simulink model "leadcar_stationary_egocar_move"  (R2025b)
settings: Solver=VariableStepAuto  StartTime=0.0  StopTime=10.0  RelTol=1e-3
settings Model: Creator=jdcjd  LastModifiedBy=jdcjd

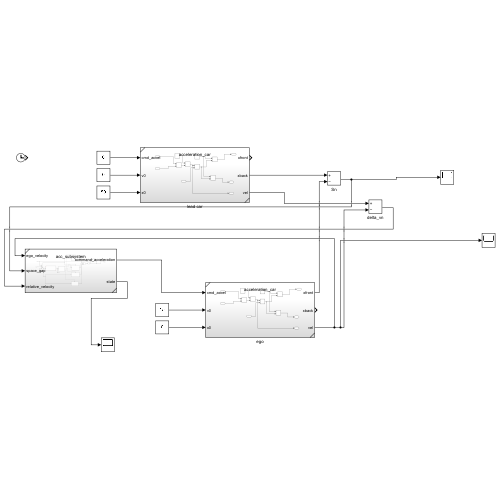
[thumbnail: Simulink's stored preview of the top-level diagram]
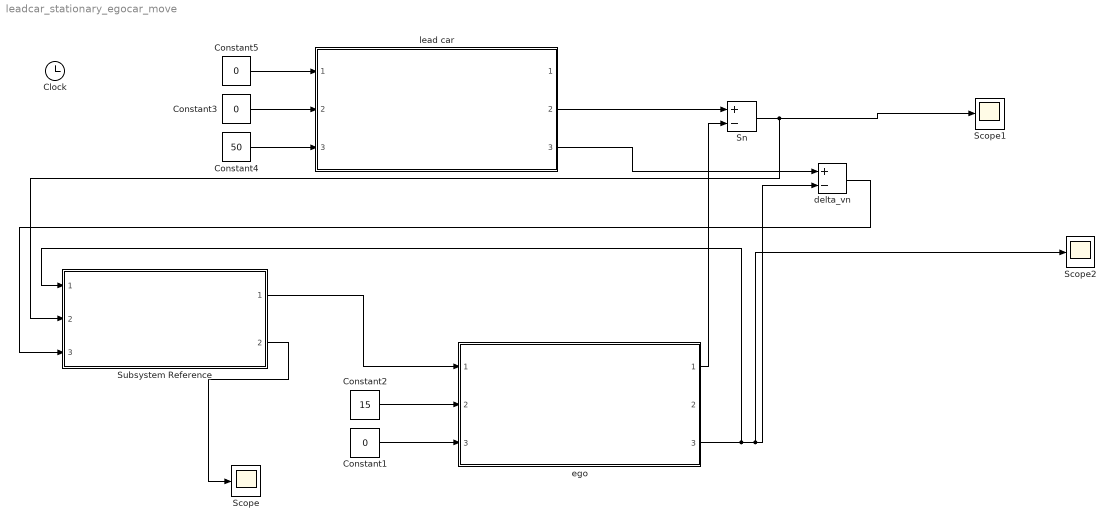
== system leadcar_stationary_egocar_move ==
  Clock : Clock
  Constant1 : Constant  Value=0
  Constant2 : Constant  Value=15
  Constant3 : Constant  Value=0
  Constant4 : Constant  Value=50
  Constant5 : Constant  Value=0
  Scope : Scope
  Scope1 : Scope
  Scope2 : Scope
      settings: DataLoggingVariableName=ScopeData2
  Sn : Sum  Inputs=+-
  Subsystem Reference : Subsystem  ReferencedSubsystem=acc_subsystem
  delta_vn : Sum  Inputs=+-
  ego : Subsystem  ReferencedSubsystem=acceleration_car
  lead car : Subsystem  ReferencedSubsystem=acceleration_car
  wires:
  Constant5/1 -> lead car/1
  Constant3/1 -> lead car/2
  Constant4/1 -> lead car/3
  Constant2/1 -> ego/2
  Constant1/1 -> ego/3
  Subsystem Reference/1 -> ego/1
  ego/1 -> Sn/2
  lead car/2 -> Sn/1
  lead car/3 -> delta_vn/1
  delta_vn/1 -> Subsystem Reference/3
  Sn/1 -> Scope1/1, Subsystem Reference/2
  Subsystem Reference/2 -> Scope/1
  ego/3 -> Subsystem Reference/1, Scope2/1, delta_vn/2
